simulink model "InterfaceModel"  (R2019b)
settings: Solver=VariableStepAuto  StartTime=0.0  StopTime=10.0  RelTol=1e-3
settings Model: Creator=sl  LastModifiedBy=a4327

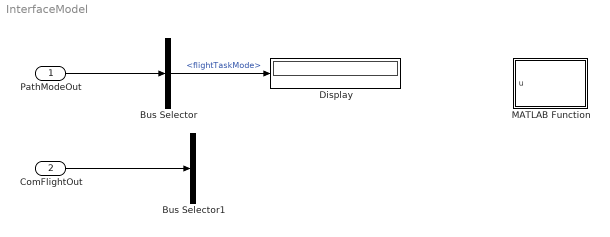
== system InterfaceModel ==
  PathModeOut : Inport  OutDataTypeStr=Bus: BUS_TASK_PATH_OutParam
  ComFlightOut : Inport  Port=2  OutDataTypeStr=Bus: BUS_TASK_COMMON_OutParam
  Bus Selector : BusSelector  OutputSignals=flightTaskMode
  Bus Selector1 : BusSelector  OutputSignals=curHomeLLA,curVelNED,curSpeed,curAirSpeed,curEuler,curWB,curPosNED,curLLA,curGroundSpeed
  Display : Display
  MATLAB Function : MATLAB Function  TreatAsAtomicUnit=on
  wires:
  PathModeOut/1 -> Bus Selector/1
  Bus Selector/1 -> Display/1  "<flightTaskMode>"
  ComFlightOut/1 -> Bus Selector1/1

== matlab function InterfaceModel/MATLAB Function ==
  data: u input
function  fcn(u)
        switch u
            %%%%%%%%%%%%%%%%%%%%%%%%%%%%%%%%%%%%%%%%%%%%%%%%%%%%%%%%%%%%%%%%%%%%%%%
            case    ENUM_FlightTaskMode.TakeOffMode
        end
